simulink model "gm_INTERLOCK_DELAY"  (R2016a)
settings: Solver=FixedStepDiscrete  StartTime=0.0  StopTime=10.0  RelTol=1e-3
libraries: simulink x12, hdlmdlgenlib x3
settings Model: Creator=zedboard  LastModifiedBy=Wendel
settings OptimizationCC: BlockReduction=off  ConditionallyExecuteInputs=off  DefaultParameterBehavior=Inlined
settings DebuggingCC: AlgebraicLoopMsg=error  InheritedTsInSrcMsg=none
settings HardwareCC: ProdBitPerPointer=32  ProdLargestAtomicFloat=None  ProdIntDivRoundTo=Undefined  ProdEndianess=Unspecified  ProdWordSize=32  ProdHWDeviceType=ASIC/FPGA->ASIC/FPGA  ProdEqTarget=off

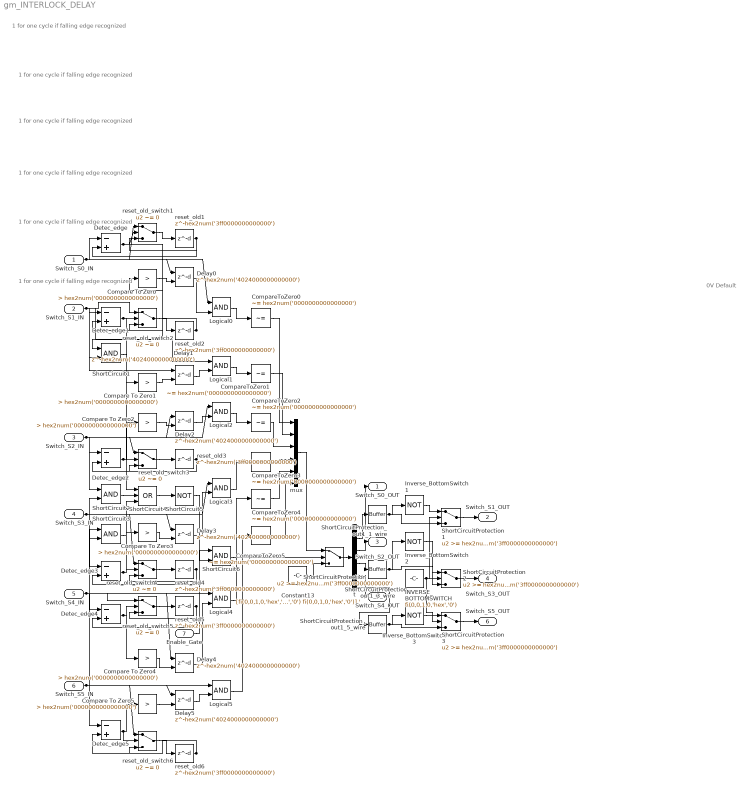
== system gm_INTERLOCK_DELAY ==
  note: 1 for one cycle if falling edge recognized
  note: 1 for one cycle if falling edge recognized
  note: 1 for one cycle if falling edge recognized
  note: 1 for one cycle if falling edge recognized
  note: 1 for one cycle if falling edge recognized
  note: 1 for one cycle if falling edge recognized
  note: 0V Default
  Switch_S0_IN : Inport  OutDataTypeStr=boolean  SampleTime=0.2
  Switch_S1_IN : Inport  Port=2  OutDataTypeStr=boolean  SampleTime=0.2
  Switch_S2_IN : Inport  Port=3  OutDataTypeStr=boolean  SampleTime=0.2
  Switch_S3_IN : Inport  Port=4  OutDataTypeStr=boolean  SampleTime=0.2
  Switch_S4_IN : Inport  Port=5  OutDataTypeStr=boolean  SampleTime=0.2
  Switch_S5_IN : Inport  Port=6  OutDataTypeStr=boolean  SampleTime=0.2
  Enable_Gate : Inport  Port=7  OutDataTypeStr=boolean  SampleTime=0.2
  Compare To Zero{,1..5} (6 alike) : simulink/Logic and Bit Operations/Compare To Constant  relop=>  const=hex2num('0000000000000000')  OutDataTypeStr=boolean
  CompareToZero{0..5} (6 alike) : simulink/Logic and Bit Operations/Compare To Constant  relop=~=  const=hex2num('0000000000000000')  OutDataTypeStr=boolean
  Constant13 : Constant  Value=[fi(0,0,1,0,'hex','0') fi(0,0,1,0,'hex','0') fi(0,0,1,0,'hex','0') fi(0,0,1,0,'hex','0') fi(0,0,1,0,'hex','0') fi(0,0,1,0,'hex','0')].'  OutDataTypeStr=boolean  SampleTime=-1
  Delay{0..5} (6 alike) : Delay  DelayLength=hex2num('4024000000000000')  InitialCondition=0  ExternalReset=Level  InputProcessing=Inherited
      settings: InputPortMap=u0,r5
  Detec_edge{,1..5} (6 alike) : Sum  Inputs=-+  AccumDataTypeStr=int8  OutDataTypeStr=int8  SampleTime=0.2
  INVERSE_BOTTOMSWITCH : Constant  Value=fi(0,0,1,0,'hex','0')  OutDataTypeStr=boolean  SampleTime=-1
  Inverse_BottomSwitch1 : Logic  Operator=NOT  Inputs=1  AllPortsSameDT=off  OutDataTypeStr=boolean  SampleTime=0.2
  Inverse_BottomSwitch2 : Logic  Operator=NOT  Inputs=1  AllPortsSameDT=off  OutDataTypeStr=boolean  SampleTime=0.2
  Inverse_BottomSwitch3 : Logic  Operator=NOT  Inputs=1  AllPortsSameDT=off  OutDataTypeStr=boolean  SampleTime=0.2
  Logical{0..5} (6 alike) : Logic  AllPortsSameDT=off  OutDataTypeStr=boolean  SampleTime=0.2
  ShortCircuit{1..3,6} (4 alike) : Logic  AllPortsSameDT=off  OutDataTypeStr=boolean  SampleTime=0.2
  ShortCircuit4 : Logic  Operator=OR  Inputs=3  AllPortsSameDT=off  OutDataTypeStr=boolean  SampleTime=0.2
  ShortCircuit5 : Logic  Operator=NOT  Inputs=1  AllPortsSameDT=off  OutDataTypeStr=boolean  SampleTime=0.2
  ShortCircuitProtection{,1..3} (4 alike) : Switch  Threshold=hex2num('3ff0000000000000')  SampleTime=0.2
  ShortCircuitProtection_out1_1_wire : hdlmdlgenlib/Buffer
  ShortCircuitProtection_out1_3_wire : hdlmdlgenlib/Buffer
  ShortCircuitProtection_out1_5_wire : hdlmdlgenlib/Buffer
  mux : Mux  Inputs=6
  reset_old{1..6} (6 alike) : Delay  DelayLength=hex2num('3ff0000000000000')  InitialCondition=0  InputProcessing=Inherited  SampleTime=0.2
  reset_old_switch{1..6} (6 alike) : Switch  Criteria=u2 ~= 0  Threshold=hex2num('0000000000000000')  SampleTime=0.2
  t : Demux  Outputs=6
  Switch_S0_OUT : Outport
  Switch_S1_OUT : Outport  Port=2
  Switch_S2_OUT : Outport  Port=3
  Switch_S3_OUT : Outport  Port=4
  Switch_S4_OUT : Outport  Port=5
  Switch_S5_OUT : Outport  Port=6
  wires:
  Switch_S0_IN/1 -> reset_old_switch1/1, ShortCircuit1/1, Logical0/1, Detec_edge/1, Delay0/1
  Switch_S1_IN/1 -> reset_old_switch2/1, ShortCircuit1/2, Logical1/1, Detec_edge1/1, Delay1/1
  Switch_S2_IN/1 -> reset_old_switch3/1, ShortCircuit2/1, Logical2/1, Detec_edge2/1, Delay2/1
  Switch_S3_IN/1 -> reset_old_switch4/1, ShortCircuit2/2, Logical3/1, Detec_edge3/1, Delay3/1
  Switch_S4_IN/1 -> reset_old_switch5/1, ShortCircuit3/1, Logical4/1, Detec_edge4/1, Delay4/1
  Switch_S5_IN/1 -> reset_old_switch6/1, ShortCircuit3/2, Logical5/1, Detec_edge5/1, Delay5/1
  Enable_Gate/1 -> ShortCircuit6/1
  Compare To Zero/1 -> Delay0/2
  Compare To Zero1/1 -> Delay1/2
  Compare To Zero2/1 -> Delay2/2
  Compare To Zero3/1 -> Delay3/2
  Compare To Zero4/1 -> Delay4/2
  Compare To Zero5/1 -> Delay5/2
  CompareToZero0/1 -> mux/1
  CompareToZero1/1 -> mux/2
  CompareToZero2/1 -> mux/3
  CompareToZero3/1 -> mux/4
  CompareToZero4/1 -> mux/5
  CompareToZero5/1 -> mux/6
  Constant13/1 -> ShortCircuitProtection/3
  Delay0/1 -> Logical0/2
  Delay1/1 -> Logical1/2
  Delay2/1 -> Logical2/2
  Delay3/1 -> Logical3/2
  Delay4/1 -> Logical4/2
  Delay5/1 -> Logical5/2
  ShortCircuitProtection_out1_1_wire/1 -> ShortCircuitProtection1/3, Inverse_BottomSwitch1/1
  ShortCircuitProtection_out1_3_wire/1 -> ShortCircuitProtection2/3, Inverse_BottomSwitch2/1
  ShortCircuitProtection_out1_5_wire/1 -> ShortCircuitProtection3/3, Inverse_BottomSwitch3/1
  Detec_edge/1 -> reset_old_switch1/2, Compare To Zero/1
  Detec_edge1/1 -> reset_old_switch2/2, Compare To Zero1/1
  Detec_edge2/1 -> reset_old_switch3/2, Compare To Zero2/1
  Detec_edge3/1 -> reset_old_switch4/2, Compare To Zero3/1
  Detec_edge4/1 -> reset_old_switch5/2, Compare To Zero4/1
  Detec_edge5/1 -> reset_old_switch6/2, Compare To Zero5/1
  INVERSE_BOTTOMSWITCH/1 -> ShortCircuitProtection3/2, ShortCircuitProtection2/2, ShortCircuitProtection1/2
  Inverse_BottomSwitch1/1 -> ShortCircuitProtection1/1
  Inverse_BottomSwitch2/1 -> ShortCircuitProtection2/1
  Inverse_BottomSwitch3/1 -> ShortCircuitProtection3/1
  Logical0/1 -> CompareToZero0/1
  Logical1/1 -> CompareToZero1/1
  Logical2/1 -> CompareToZero2/1
  Logical3/1 -> CompareToZero3/1
  Logical4/1 -> CompareToZero4/1
  Logical5/1 -> CompareToZero5/1
  mux/1 -> ShortCircuitProtection/1
  ShortCircuit1/1 -> ShortCircuit4/1
  ShortCircuit2/1 -> ShortCircuit4/2
  ShortCircuit3/1 -> ShortCircuit4/3
  ShortCircuit4/1 -> ShortCircuit5/1
  ShortCircuit5/1 -> ShortCircuit6/2
  ShortCircuit6/1 -> ShortCircuitProtection/2
  ShortCircuitProtection/1 -> t/1
  ShortCircuitProtection1/1 -> Switch_S1_OUT/1
  ShortCircuitProtection2/1 -> Switch_S3_OUT/1
  ShortCircuitProtection3/1 -> Switch_S5_OUT/1
  reset_old1/1 -> reset_old_switch1/3, Detec_edge/2
  reset_old2/1 -> reset_old_switch2/3, Detec_edge1/2
  reset_old3/1 -> reset_old_switch3/3, Detec_edge2/2
  reset_old4/1 -> reset_old_switch4/3, Detec_edge3/2
  reset_old5/1 -> reset_old_switch5/3, Detec_edge4/2
  reset_old6/1 -> reset_old_switch6/3, Detec_edge5/2
  reset_old_switch1/1 -> reset_old1/1
  reset_old_switch2/1 -> reset_old2/1
  reset_old_switch3/1 -> reset_old3/1
  reset_old_switch4/1 -> reset_old4/1
  reset_old_switch5/1 -> reset_old5/1
  reset_old_switch6/1 -> reset_old6/1
  t/1 -> Switch_S0_OUT/1
  t/2 -> ShortCircuitProtection_out1_1_wire/1
  t/3 -> Switch_S2_OUT/1
  t/4 -> ShortCircuitProtection_out1_3_wire/1
  t/5 -> Switch_S4_OUT/1
  t/6 -> ShortCircuitProtection_out1_5_wire/1
